simulink model "VHF_AM"  (R2023b)
settings: Solver=FixedStepAuto  StartTime=0.0  StopTime=0.004  FixedStep=1/(2*244500000)  RelTol=1e-3
undefined symbols (not defined in the file or in its folder): dfilt
libraries: dsparch4 x3, simulink x1
settings Model: Creator=86134  LastModifiedBy=86134
settings OptimizationCC: ReuseModelBlockBuffer=off

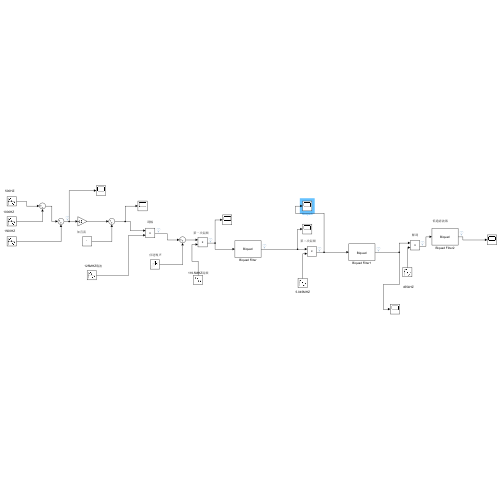
[thumbnail: Simulink's stored preview of the top-level diagram]
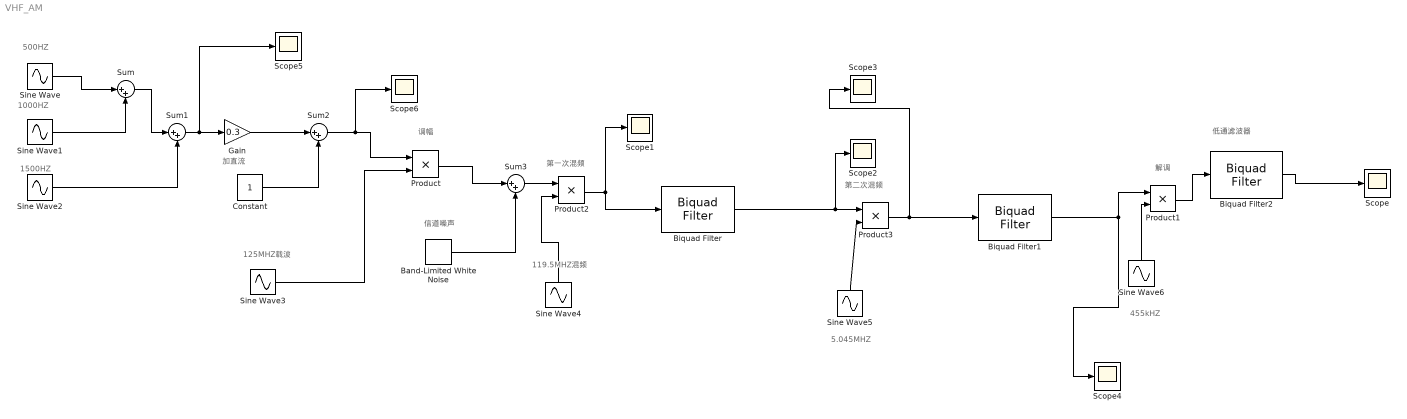
== system VHF_AM ==
  note: 455kHZ
  note: 低通滤波器
  note: 第二次混频
  note: 解调
  note: 5.045MHZ
  note: 119.5MHZ混频
  note: 信道噪声
  note: 调幅
  note: 125MHZ载波
  note: 加直流
  note: 1500HZ
  note: 1000HZ
  note: 500HZ
  note: 第一次混频
  Band-Limited White Noise : simulink/Sources/Band-Limited White Noise  Cov=0.01  Ts=1/(2*244500000)  seed=[23341]
  Biquad Filter : dsparch4/Biquad Filter  FilterSource=Dialog parameters  CoeffSource=Specify via dialog  FilterObject=dfilt.df2tsos([1 0.3 0.4],[1 0.1 0.2])  IIRFiltStruct=Direct form II transposed  BiQuadCoeffs=[9.986658649379e-05 0 -9.986658649379e-05 1 -1.99498016496809 0.999986350492765;9.986658649379e-05 0 -9.986658649379e-05 1 -1.99500834404606 0.999986388959867;9.98652379997611e-05 0 -9.98652379997611e-05 1 -1.99495345248758 0.999959307528256;9.98652379997611e-05 0 -9.98652379997611e-05 1 -1.99498118062253 0.999959419739473;9.98639273560039e-05 0 -9.98639273560039e-05 1 -1.99492775777253 0.999933026345481;9.98639273560039e-05 0 -9.98639273560039e-05 1 -1.99495451234916 0.999933204082068;9.98626789714586e-05 0 -9.98626789714586e-05 1 -1.99490356119255 0.999907998243975;9.98626789714586e-05 0 -9.98626789714586e-05 1 -1.99492883396688 0.999908228448088;9.98615160929089e-05 0 -9.98615160929089e-05 1 -1.99488131479193 0.99988469100264;9.98615160929089e-05 0 -9.98615160929089e-05 1 -1.99490462206761 0.999884956313077;9.98604603725504e-05 0 -9.98604603725504e-05 1 -1.99486143326856 0.999863539220061;9.98604603725504e-05 0 -9.98604603725504e-05 1 -1.99488232684931 0.999863820496247;9.98595314653956e-05 0 -9.98595314653956e-05 1 -1.9948442874466 0.999844937557527;9.98595314653956e-05 0 -9.98595314653956e-05 1 -1.99486236257154 0.999845213778944;9.9858746663958e-05 0 -9.9858746663958e-05 1 -1.99483019654399 0.999829232361145;9.9858746663958e-05 0 -9.9858746663958e-05 1 -1.99484510070701 0.999829482635879;9.98581205769612e-05 0 -9.98581205769612e-05 1 -1.99481942146171 0.999816715107375;9.98581205769612e-05 0 -9.98581205769612e-05 1 -1.99483086383058 0.99981692090596;9.98576648579943e-05 0 -9.98576648579943e-05 1 -1.99481216214234 0.999807617623362;9.98576648579943e-05 0 -9.98576648579943e-05 1 -1.99481991743367 0.999807763689727;9.98573879891126e-05 0 -9.98573879891126e-05 1 -1.99480855145785 0.999802108013933;9.98573879891126e-05 0 -9.98573879891126e-05 1 -1.99481246740269 0.99980218274255;9.98572951233601e-05 0 -9.98572951233601e-05 1 -1.99480865447323 0.999800285409753]  ScaleValues=1  IC=0  ICnum=0  ICden=0  a0Flag=Warning  optimizeScaleValues=on  ScaleValueMode=Specify via input port (g)  roundingMode=Floor  overflowMode=off  scaleValueFracLength=14  denProdOutputFracLength=30  denAccumFracLength=30  secondMemoryFracLength=15
      settings: LibrarySourceBlock=dsphdlsupportfiltering/Biquad Filter
  Biquad Filter1 : dsparch4/Biquad Filter  FilterSource=Dialog parameters  CoeffSource=Specify via dialog  FilterObject=dfilt.df2tsos([1 0.3 0.4],[1 0.1 0.2])  IIRFiltStruct=Direct form II transposed  BiQuadCoeffs=[4.03948489928381e-05 0 -4.03948489928381e-05 1 -1.99995684514404 0.999991494438868;4.03948489928381e-05 0 -4.03948489928381e-05 1 -1.99995790335016 0.999991615915197;4.03945153254835e-05 0 -4.03945153254835e-05 1 -1.99994024021482 0.999974869803924;4.03945153254835e-05 0 -4.03945153254835e-05 1 -1.99994146867516 0.999975199829275;4.03942037027879e-05 0 -4.03942037027879e-05 1 -1.99992477629048 0.999959362842132;4.03942037027879e-05 0 -4.03942037027879e-05 1 -1.99992607609482 0.999959848750576;4.03939277421844e-05 0 -4.03939277421844e-05 1 -1.99991113661551 0.999945665808666;4.03939277421844e-05 0 -4.03939277421844e-05 1 -1.99991239068134 0.999946218938011;4.03936995019497e-05 0 -4.03936995019497e-05 1 -1.99989991731187 0.999934370480905;4.03936995019497e-05 0 -4.03936995019497e-05 1 -1.99990101021673 0.99993491276175;4.0393528954636e-05 0 -4.0393528954636e-05 1 -1.99989161756128 0.999925981423023;4.0393528954636e-05 0 -4.0393528954636e-05 1 -1.99989242288893 0.999926413277462;4.03934235516796e-05 0 -4.03934235516796e-05 1 -1.99988658939949 0.999920858598401;4.03934235516796e-05 0 -4.03934235516796e-05 1 -1.99988701440491 0.999921098480289;4.03933878981345e-05 0 -4.03933878981345e-05 1 -1.99988503675829 0.999919213224204]  ScaleValues=1  IC=0  ICnum=0  ICden=0  a0Flag=Warning  optimizeScaleValues=on  ScaleValueMode=Specify via input port (g)  roundingMode=Floor  overflowMode=off  scaleValueFracLength=14  denProdOutputFracLength=30  denAccumFracLength=30  secondMemoryFracLength=15
      settings: LibrarySourceBlock=dsphdlsupportfiltering/Biquad Filter
  Biquad Filter2 : dsparch4/Biquad Filter  FilterSource=Dialog parameters  CoeffSource=Specify via dialog  FilterObject=dfilt.df2tsos([1 0.3 0.4],[1 0.1 0.2])  IIRFiltStruct=Direct form II transposed  BiQuadCoeffs=[8.67983807175607e-10 1.73596761435121e-09 8.67983807175607e-10 1 -1.99999512654035 0.999995130012286;8.67979594563164e-10 1.73595918912633e-09 8.67979594563164e-10 1 -1.99998541990264 0.999985423374557;8.67975425204918e-10 1.73595085040984e-09 8.67975425204918e-10 1 -1.99997581293059 0.999975816402492;8.67971327580159e-10 1.73594265516032e-09 8.67971327580159e-10 1 -1.99996637124576 0.999966374717643;8.67967329677399e-10 1.7359346593548e-09 8.67967329677399e-10 1 -1.99995715933884 0.999957162810709;8.6796345880324e-10 1.73592691760648e-09 8.6796345880324e-10 1 -1.9999482401293 0.999948243601156;8.67959741395936e-10 1.73591948279187e-09 8.67959741395936e-10 1 -1.99993967453576 0.9999396780076;8.67956202844886e-10 1.73591240568977e-09 8.67956202844886e-10 1 -1.99993152106009 0.999931524531915;8.67952867317324e-10 1.73590573463465e-09 8.67952867317324e-10 1 -1.99992383538806 0.999923838859873;8.67949757593353e-10 1.73589951518671e-09 8.67949757593353e-10 1 -1.99991667000924 0.999916673481041;8.67946894910469e-10 1.73589378982094e-09 8.67946894910469e-10 1 -1.99991007385875 0.999910077330538;8.6794429881863e-10 1.73588859763726e-09 8.6794429881863e-10 1 -1.9999040919833 0.999904095455078;8.67941987046842e-10 1.73588397409368e-09 8.67941987046842e-10 1 -1.9998987652338 0.999898768705571;8.67939975382192e-10 1.73587995076438e-09 8.67939975382192e-10 1 -1.99989412998662 0.999894133458382;8.67938277562131e-10 1.73587655512426e-09 8.67938277562131e-10 1 -1.99989021789538 0.999890221367135;8.67936905180747e-10 1.73587381036149e-09 8.67936905180747e-10 1 -1.99988705567501 0.999887059146755;8.67935867609673e-10 1.73587173521935e-09 8.67935867609673e-10 1 -1.99988466491947 0.999884668391216;8.6793517193415e-10 1.7358703438683e-09 8.6793517193415e-10 1 -1.99988306195448 0.999883065426221;8.67934822904694e-10 1.73586964580939e-09 8.67934822904694e-10 1 -1.9998822577261 0.99988226119784]  ScaleValues=1  IC=0  ICnum=0  ICden=0  a0Flag=Warning  optimizeScaleValues=on  ScaleValueMode=Specify via input port (g)  roundingMode=Floor  overflowMode=off  scaleValueFracLength=14  denProdOutputFracLength=30  denAccumFracLength=30  secondMemoryFracLength=15
      settings: LibrarySourceBlock=dsphdlsupportfiltering/Biquad Filter
  Constant : Constant
  Gain : Gain  Gain=0.3
  Product{,1..3} (4 alike) : Product
  Scope{,1..6} (7 alike) : Scope
  Sine Wave : Sin  Frequency=500*2*pi  SampleTime=0
  Sine Wave1 : Sin  Frequency=1000*2*pi  SampleTime=0
  Sine Wave2 : Sin  Frequency=1500*2*pi  SampleTime=0
  Sine Wave3 : Sin  Frequency=125000000*2*pi  SampleTime=0
  Sine Wave4 : Sin  Frequency=119500000*2*pi  SampleTime=0
  Sine Wave5 : Sin  Frequency=5045000*2*pi  SampleTime=0
  Sine Wave6 : Sin  Frequency=455000*2*pi  SampleTime=0
  Sum{,1..3} (4 alike) : Sum  Inputs=|++
  wires:
  Sine Wave/1 -> Sum/1
  Sine Wave1/1 -> Sum/2
  Sum/1 -> Sum1/1
  Sine Wave2/1 -> Sum1/2
  Sum1/1 -> Scope5/1, Gain/1
  Gain/1 -> Sum2/1
  Constant/1 -> Sum2/2
  Sum2/1 -> Scope6/1, Product/1
  Sine Wave3/1 -> Product/2
  Product/1 -> Sum3/1
  Band-Limited White Noise/1 -> Sum3/2
  Sum3/1 -> Product2/1
  Sine Wave4/1 -> Product2/2
  Sine Wave5/1 -> Product3/2
  Biquad Filter/1 -> Scope2/1, Product3/1
  Product3/1 -> Biquad Filter1/1, Scope3/1
  Sine Wave6/1 -> Product1/2
  Biquad Filter1/1 -> Product1/1, Scope4/1
  Product2/1 -> Biquad Filter/1, Scope1/1
  Product1/1 -> Biquad Filter2/1
  Biquad Filter2/1 -> Scope/1
